simulink subsystem "test_actuation_system"  (R2021a)
settings: Solver=VariableStepAuto  StartTime=0.0  StopTime=10.0  RelTol=1e-3
libraries: sm_lib x51, nesl_utility x5
settings Model: Creator=Daniel Adejumo  LastModifiedBy=Daniel Adejumo

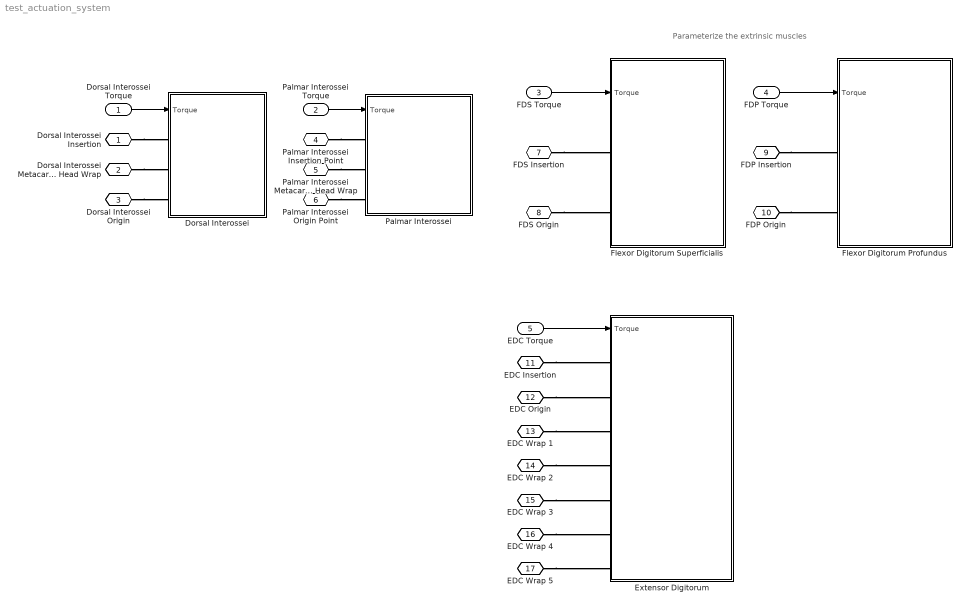
== system test_actuation_system ==
  note: Parameterize the extrinsic muscles
  Dorsal Interossei Torque : Inport
  Palmar Interossei Torque : Inport  Port=2
  FDS Torque : Inport  Port=3
  FDP Torque : Inport  Port=4
  EDC Torque : Inport  Port=5
  Dorsal Interossei : Subsystem
  Extensor Digitorum : Subsystem
  Flexor Digitorum Profundus : Subsystem
  Flexor Digitorum Superficialis : Subsystem
  Palmar Interossei : Subsystem
  Dorsal Interossei Insertion : PMIOPort  Side=Left
  Dorsal Interossei Metacarpal Head Wrap : PMIOPort  Port=2  Side=Left
  Dorsal Interossei Origin : PMIOPort  Port=3  Side=Left
  Palmar Interossei Insertion Point : PMIOPort  Port=4  Side=Left
  Palmar Interossei Metacarpal Head Wrap : PMIOPort  Port=5  Side=Left
  Palmar Interossei Origin Point : PMIOPort  Port=6  Side=Left
  FDS Insertion : PMIOPort  Port=7  Side=Left
  FDS Origin : PMIOPort  Port=8  Side=Left
  FDP Insertion : PMIOPort  Port=9  Side=Left
  FDP Origin : PMIOPort  Port=10  Side=Left
  EDC Insertion : PMIOPort  Port=11  Side=Left
  EDC Origin : PMIOPort  Port=12  Side=Left
  EDC Wrap 1 : PMIOPort  Port=13  Side=Left
  EDC Wrap 2 : PMIOPort  Port=14  Side=Left
  EDC Wrap 3 : PMIOPort  Port=15  Side=Left
  EDC Wrap 4 : PMIOPort  Port=16  Side=Left
  EDC Wrap 5 : PMIOPort  Port=17  Side=Left
  wires:
  Dorsal Interossei Torque/1 -> Dorsal Interossei/1(Torque)
  Palmar Interossei Torque/1 -> Palmar Interossei/1(Torque)
  FDS Torque/1 -> Flexor Digitorum Superficialis/1(Torque)
  FDP Torque/1 -> Flexor Digitorum Profundus/1(Torque)
  EDC Torque/1 -> Extensor Digitorum/1(Torque)
  connections:
  Dorsal Interossei Insertion/RConn1 -- Dorsal Interossei/LConn1
  Dorsal Interossei Metacarpal Head Wrap/RConn1 -- Dorsal Interossei/LConn2
  Dorsal Interossei Origin/RConn1 -- Dorsal Interossei/LConn3
  Palmar Interossei Insertion Point/RConn1 -- Palmar Interossei/LConn1
  FDS Insertion/RConn1 -- Flexor Digitorum Superficialis/LConn1
  FDS Origin/RConn1 -- Flexor Digitorum Superficialis/LConn2
  Palmar Interossei Metacarpal Head Wrap/RConn1 -- Palmar Interossei/LConn2
  Palmar Interossei Origin Point/RConn1 -- Palmar Interossei/LConn3
  FDP Origin/RConn1 -- Flexor Digitorum Profundus/LConn2
  FDP Insertion/RConn1 -- Flexor Digitorum Profundus/LConn1
  EDC Insertion/RConn1 -- Extensor Digitorum/LConn1
  EDC Origin/RConn1 -- Extensor Digitorum/LConn2
  EDC Wrap 1/RConn1 -- Extensor Digitorum/LConn3
  EDC Wrap 2/RConn1 -- Extensor Digitorum/LConn4
  EDC Wrap 3/RConn1 -- Extensor Digitorum/LConn5
  EDC Wrap 4/RConn1 -- Extensor Digitorum/LConn6
  EDC Wrap 5/RConn1 -- Extensor Digitorum/LConn7

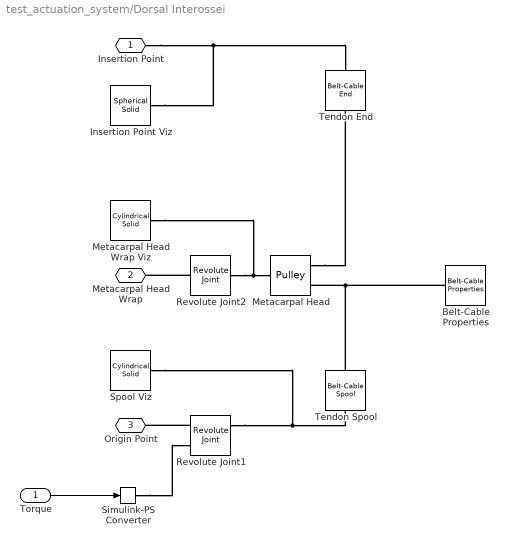
== system test_actuation_system/Dorsal Interossei ==
  Torque : Inport
  Belt-Cable Properties : sm_lib/Belts and Cables/Belt-Cable Properties  DrumBeltCableAlignment=Unrestricted  GraphicType=PitchLine  GraphicVisPropType=SimpleVisualProperties  GraphicDiffuseColor=viz.d2.dorsal_interossei.tendon_color  GraphicSpecularColor=[0.5 0.5 0.5 1.0]  GraphicAmbientColor=[0.15 0.15 0.15 1.0]  GraphicEmissiveColor=[0.0 0.0 0.0 1.0]  GraphicShininess=75  GraphicOpacity=viz.d2.dorsal_interossei.tendon_opacity
      settings: SourceProductBaseCode=MS
  Insertion Point Viz : sm_lib/Body Elements/Spherical Solid  GraphicAmbientColor=[0.15 0.15 0.15 1.0]  BasedOnType=Density  CenterOfMass=[0 0 0]  CenterOfMassUnits=m  GraphicDiffuseColor=viz.d2.dorsal_interossei.insertion_point_color  Density=dnm.link_density  DensityUnits=kg/m^3  DoExposeReferenceFrame=on  GraphicEmissiveColor=[0.0 0.0 0.0 1.0]  ExportEntireGeometry=off  SerializedExposedGeometries=<ExposedGeometries/>  SerializedFrames=<Frames/>  MarkerShape=Sphere  MarkerSize=10  GraphicType=FromGeometry  InertiaType=CalculateFromGeometry  Mass=1  MassUnits=kg  MomentsOfInertia=[1 1 1]  MomentsOfInertiaUnits=kg*m^2  GraphicOpacity=viz.d2.dorsal_interossei.insertion_point_opacity  ProductsOfInertia=[0 0 0]  ProductsOfInertiaUnits=kg*m^2  GraphicShininess=75  GraphicSpecularColor=[0.5 0.5 0.5 1.0]  SphereRadius=viz.d2.dorsal_interossei.insertion_point_radius  SphereRadiusUnits=m  GraphicVisPropType=SimpleVisualProperties
  Metacarpal Head : sm_lib/Belts and Cables/Pulley  PitchRadius=knm.d2.dorsal_interossei.wrap_pulleys_radius  PitchRadiusUnits=m  InitialWrapAngleLowerBound=knm.d2.dorsal_interossei.initial_wrap_lower_bound  InitialWrapAngleLowerBoundUnits=deg  SenseWrapAngle=off  SensePulleyAngleA=off  SensePulleyAngleB=off  SenseFleetAngleA=off  SenseFleetAngleB=off
      settings: SourceProductBaseCode=MS
  Metacarpal Head Wrap Viz : sm_lib/Body Elements/Cylindrical Solid  GraphicAmbientColor=[0.15 0.15 0.15 1.0]  BasedOnType=Density  CenterOfMass=[0 0 0]  CenterOfMassUnits=m  GraphicDiffuseColor=viz.d2.dorsal_interossei.wrap_pulleys_color  CylinderLength=viz.d2.dorsal_interossei.wrap_pulleys_length  CylinderLengthUnits=m  CylinderRadius=knm.d2.dorsal_interossei.wrap_pulleys_radius  CylinderRadiusUnits=m  Density=dnm.link_density  DensityUnits=kg/m^3  DoExposeReferenceFrame=on  GraphicEmissiveColor=[0.0 0.0 0.0 1.0]  ExportEntireGeometry=off  SerializedFrames=<Frames/>  MarkerShape=Sphere  MarkerSize=10  GraphicType=FromGeometry  InertiaType=CalculateFromGeometry  Mass=1  MassUnits=kg  MomentsOfInertia=[1 1 1]  MomentsOfInertiaUnits=kg*m^2  GraphicOpacity=viz.d2.dorsal_interossei.wrap_pulleys_opacity  ProductsOfInertia=[0 0 0]  ProductsOfInertiaUnits=kg*m^2  GraphicShininess=75  GraphicSpecularColor=[0.5 0.5 0.5 1.0]  GraphicVisPropType=SimpleVisualProperties
  Revolute Joint1 : sm_lib/Joints/Revolute Joint  JointMode=Normal  SenseConstraintForce=off  SenseConstraintForceX=off  SenseConstraintForceY=off  SenseConstraintForceZ=off  SenseConstraintTorque=off  SenseConstraintTorqueX=off  SenseConstraintTorqueY=off  SenseConstraintTorqueZ=off  SenseTotalForce=off  SenseTotalForceX=off  SenseTotalForceY=off  SenseTotalForceZ=off  SenseTotalTorque=off  SenseTotalTorqueX=off  SenseTotalTorqueY=off  SenseTotalTorqueZ=off  CompositeWrenchDir=FollowerOnBase  CompositeWrenchFrame=BaseFrame  EquilibriumPosition=0  EquilibriumPositionUnits=deg  SpringStiffness=0  SpringStiffnessUnits=N*m/deg  DampingCoefficient=0  DampingCoefficientUnits=N*m/(deg/s)  TorqueActuationMode=InputTorque  MotionActuationMode=ComputedMotion  SensePosition=off  SenseVelocity=on  SenseAcceleration=off  SenseTorqueForce=off  SenseLowerLimitTorqueForce=off  SenseUpperLimitTorqueForce=off  LowerLimitSpecify=off  LowerLimitBound=-90  LowerLimitBoundUnits=deg  LowerLimitStiffness=1e4  LowerLimitStiffnessUnits=N*m/deg  LowerLimitDamping=10  LowerLimitDampingUnits=N*m/(deg/s)  LowerLimitTransitionRegionWidth=0.1  LowerLimitTransitionRegionWidthUnits=deg  UpperLimitSpecify=off  UpperLimitBound=90  UpperLimitBoundUnits=deg  UpperLimitStiffness=1e4  UpperLimitStiffnessUnits=N*m/deg  UpperLimitDamping=10  UpperLimitDampingUnits=N*m/(deg/s)  UpperLimitTransitionRegionWidth=0.1  UpperLimitTransitionRegionWidthUnits=deg  PositionTargetSpecify=off  PositionTargetPriority=High  PositionTargetValue=0  PositionTargetValueUnits=deg  VelocityTargetSpecify=off  VelocityTargetPriority=High  VelocityTargetValue=0  VelocityTargetValueUnits=deg/s
  Revolute Joint2 : sm_lib/Joints/Revolute Joint  JointMode=Normal  SenseConstraintForce=off  SenseConstraintForceX=off  SenseConstraintForceY=off  SenseConstraintForceZ=off  SenseConstraintTorque=off  SenseConstraintTorqueX=off  SenseConstraintTorqueY=off  SenseConstraintTorqueZ=off  SenseTotalForce=off  SenseTotalForceX=off  SenseTotalForceY=off  SenseTotalForceZ=off  SenseTotalTorque=off  SenseTotalTorqueX=off  SenseTotalTorqueY=off  SenseTotalTorqueZ=off  CompositeWrenchDir=FollowerOnBase  CompositeWrenchFrame=BaseFrame  EquilibriumPosition=0  EquilibriumPositionUnits=deg  SpringStiffness=0  SpringStiffnessUnits=N*m/deg  DampingCoefficient=0  DampingCoefficientUnits=N*m/(deg/s)  TorqueActuationMode=NoTorque  MotionActuationMode=ComputedMotion  SensePosition=off  SenseVelocity=off  SenseAcceleration=off  SenseTorqueForce=off  SenseLowerLimitTorqueForce=off  SenseUpperLimitTorqueForce=off  LowerLimitSpecify=off  LowerLimitBound=-90  LowerLimitBoundUnits=deg  LowerLimitStiffness=1e4  LowerLimitStiffnessUnits=N*m/deg  LowerLimitDamping=10  LowerLimitDampingUnits=N*m/(deg/s)  LowerLimitTransitionRegionWidth=0.1  LowerLimitTransitionRegionWidthUnits=deg  UpperLimitSpecify=off  UpperLimitBound=90  UpperLimitBoundUnits=deg  UpperLimitStiffness=1e4  UpperLimitStiffnessUnits=N*m/deg  UpperLimitDamping=10  UpperLimitDampingUnits=N*m/(deg/s)  UpperLimitTransitionRegionWidth=0.1  UpperLimitTransitionRegionWidthUnits=deg  PositionTargetSpecify=off  PositionTargetPriority=High  PositionTargetValue=0  PositionTargetValueUnits=deg  VelocityTargetSpecify=off  VelocityTargetPriority=High  VelocityTargetValue=0  VelocityTargetValueUnits=deg/s
  Simulink-PS Converter : nesl_utility/Simulink-PS Converter  PhysicalDomain=network_engine_domain  SubClassName=ps_input  LeftPortType=input  RightPortType=output  PseudoPeriodic=off  Frequencies=[]  NoiseDistribution=none  NoiseParameters=[]  Unit=N*m  AffineConversion=off  FilteringAndDerivatives=filter  SimscapeFilterOrder=2  InputFilterTimeConstant=0.001  UdotUserProvided=0
      settings: SourceProductBaseCode=PW,SS
  Spool Viz : sm_lib/Body Elements/Cylindrical Solid  GraphicAmbientColor=[0.15 0.15 0.15 1.0]  BasedOnType=Density  CenterOfMass=[0 0 0]  CenterOfMassUnits=m  GraphicDiffuseColor=viz.d2.dorsal_interossei.spool_color  CylinderLength=viz.d2.dorsal_interossei.spool_length  CylinderLengthUnits=m  CylinderRadius=knm.d2.dorsal_interossei.pitch_radius  CylinderRadiusUnits=m  Density=dnm.link_density  DensityUnits=kg/m^3  DoExposeReferenceFrame=on  GraphicEmissiveColor=[0.0 0.0 0.0 1.0]  ExportEntireGeometry=off  SerializedFrames=<Frames/>  MarkerShape=Sphere  MarkerSize=10  GraphicType=FromGeometry  InertiaType=CalculateFromGeometry  Mass=1  MassUnits=kg  MomentsOfInertia=[1 1 1]  MomentsOfInertiaUnits=kg*m^2  GraphicOpacity=viz.d2.dorsal_interossei.spool_opacity  ProductsOfInertia=[0 0 0]  ProductsOfInertiaUnits=kg*m^2  GraphicShininess=75  GraphicSpecularColor=[0.5 0.5 0.5 1.0]  GraphicVisPropType=SimpleVisualProperties
  Tendon End : sm_lib/Belts and Cables/Belt-Cable End
      settings: SourceProductBaseCode=MS
  Tendon Spool : sm_lib/Belts and Cables/Belt-Cable Spool  PitchRadius=knm.d2.dorsal_interossei.pitch_radius  PitchRadiusUnits=m  SenseSpoolAngleA=off  SenseFleetAngleA=off
      settings: SourceProductBaseCode=MS
  Insertion Point : PMIOPort  Side=Left
  Metacarpal Head Wrap : PMIOPort  Port=2  Side=Left
  Origin Point : PMIOPort  Port=3  Side=Left
  wires:
  Torque/1 -> Simulink-PS Converter/1
  connections:
  Simulink-PS Converter/RConn1 -- Revolute Joint1/LConn2
  Metacarpal Head Wrap Viz/RConn1 -- Revolute Joint2/RConn1 -- Metacarpal Head/LConn1
  Revolute Joint2/LConn1 -- Metacarpal Head Wrap/RConn1
  Spool Viz/RConn1 -- Revolute Joint1/RConn1 -- Tendon Spool/LConn1
  Metacarpal Head/RConn1 -- Tendon End/RConn1
  Revolute Joint1/LConn1 -- Origin Point/RConn1
  Belt-Cable Properties/LConn1 -- Tendon Spool/RConn1 -- Metacarpal Head/RConn2
  Insertion Point Viz/RConn1 -- Insertion Point/RConn1 -- Tendon End/LConn1

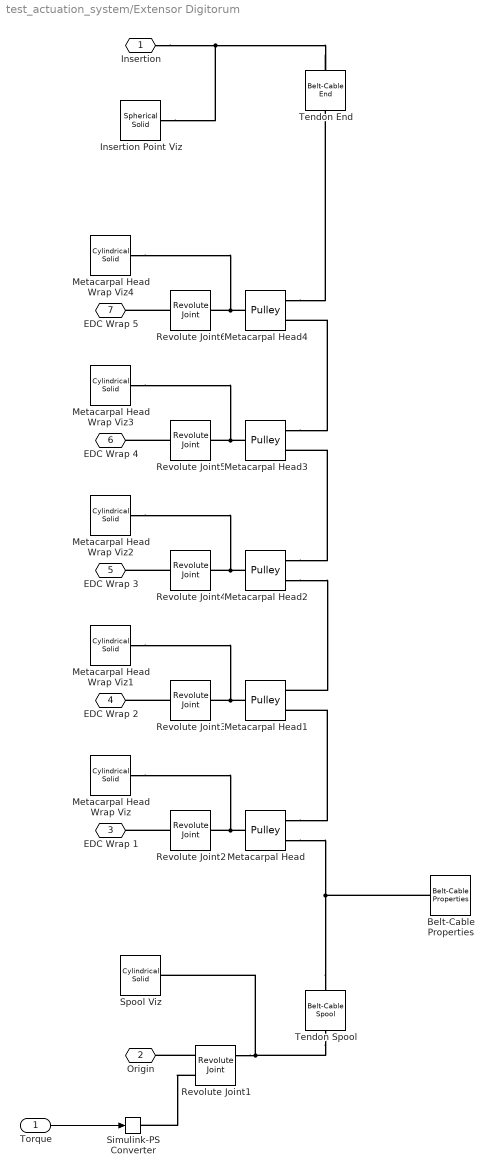
== system test_actuation_system/Extensor Digitorum ==
  Torque : Inport
  Belt-Cable Properties : sm_lib/Belts and Cables/Belt-Cable Properties  DrumBeltCableAlignment=Unrestricted  GraphicType=PitchLine  GraphicVisPropType=SimpleVisualProperties  GraphicDiffuseColor=viz.d2.palmar_interossei.tendon_color  GraphicSpecularColor=[0.5 0.5 0.5 1.0]  GraphicAmbientColor=[0.15 0.15 0.15 1.0]  GraphicEmissiveColor=[0.0 0.0 0.0 1.0]  GraphicShininess=75  GraphicOpacity=viz.d2.palmar_interossei.wrap_pulleys_opacity
      settings: SourceProductBaseCode=MS
  Insertion Point Viz : sm_lib/Body Elements/Spherical Solid  GraphicAmbientColor=[0.15 0.15 0.15 1.0]  BasedOnType=Density  CenterOfMass=[0 0 0]  CenterOfMassUnits=m  GraphicDiffuseColor=viz.d2.palmar_interossei.insertion_point_color  Density=1000  DensityUnits=kg/m^3  DoExposeReferenceFrame=on  GraphicEmissiveColor=[0.0 0.0 0.0 1.0]  ExportEntireGeometry=off  SerializedExposedGeometries=<ExposedGeometries/>  SerializedFrames=<Frames/>  MarkerShape=Sphere  MarkerSize=10  GraphicType=FromGeometry  InertiaType=CalculateFromGeometry  Mass=1  MassUnits=kg  MomentsOfInertia=[1 1 1]  MomentsOfInertiaUnits=kg*m^2  GraphicOpacity=viz.d2.palmar_interossei.insertion_point_opacity  ProductsOfInertia=[0 0 0]  ProductsOfInertiaUnits=kg*m^2  GraphicShininess=75  GraphicSpecularColor=[0.5 0.5 0.5 1.0]  SphereRadius=viz.d2.palmar_interossei.insertion_point_radius  SphereRadiusUnits=m  GraphicVisPropType=SimpleVisualProperties
  Metacarpal Head{,1..4} (5 alike) : sm_lib/Belts and Cables/Pulley  PitchRadius=knm.d2.palmar_interossei.wrap_pulleys_radius  PitchRadiusUnits=m  InitialWrapAngleLowerBound=knm.d2.palmar_interossei.initial_wrap_lower_bound  InitialWrapAngleLowerBoundUnits=deg  SenseWrapAngle=off  SensePulleyAngleA=off  SensePulleyAngleB=off  SenseFleetAngleA=off  SenseFleetAngleB=off
      settings: SourceProductBaseCode=MS
  Metacarpal Head Wrap Viz{,1..4} (5 alike) : sm_lib/Body Elements/Cylindrical Solid  GraphicAmbientColor=[0.15 0.15 0.15 1.0]  BasedOnType=Density  CenterOfMass=[0 0 0]  CenterOfMassUnits=m  GraphicDiffuseColor=viz.d2.palmar_interossei.wrap_pulleys_color  CylinderLength=viz.d2.palmar_interossei.wrap_pulleys_length  CylinderLengthUnits=m  CylinderRadius=knm.d2.palmar_interossei.wrap_pulleys_radius  CylinderRadiusUnits=m  Density=dnm.link_density  DensityUnits=kg/m^3  DoExposeReferenceFrame=on  GraphicEmissiveColor=[0.0 0.0 0.0 1.0]  ExportEntireGeometry=off  SerializedFrames=<Frames/>  MarkerShape=Sphere  MarkerSize=10  GraphicType=FromGeometry  InertiaType=CalculateFromGeometry  Mass=1  MassUnits=kg  MomentsOfInertia=[1 1 1]  MomentsOfInertiaUnits=kg*m^2  GraphicOpacity=viz.d2.palmar_interossei.wrap_pulleys_opacity  ProductsOfInertia=[0 0 0]  ProductsOfInertiaUnits=kg*m^2  GraphicShininess=75  GraphicSpecularColor=[0.5 0.5 0.5 1.0]  GraphicVisPropType=SimpleVisualProperties
  Revolute Joint1 : sm_lib/Joints/Revolute Joint  JointMode=Normal  SenseConstraintForce=off  SenseConstraintForceX=off  SenseConstraintForceY=off  SenseConstraintForceZ=off  SenseConstraintTorque=off  SenseConstraintTorqueX=off  SenseConstraintTorqueY=off  SenseConstraintTorqueZ=off  SenseTotalForce=off  SenseTotalForceX=off  SenseTotalForceY=off  SenseTotalForceZ=off  SenseTotalTorque=off  SenseTotalTorqueX=off  SenseTotalTorqueY=off  SenseTotalTorqueZ=off  CompositeWrenchDir=FollowerOnBase  CompositeWrenchFrame=BaseFrame  EquilibriumPosition=0  EquilibriumPositionUnits=deg  SpringStiffness=0  SpringStiffnessUnits=N*m/deg  DampingCoefficient=0  DampingCoefficientUnits=N*m/(deg/s)  TorqueActuationMode=InputTorque  MotionActuationMode=ComputedMotion  SensePosition=off  SenseVelocity=on  SenseAcceleration=off  SenseTorqueForce=off  SenseLowerLimitTorqueForce=off  SenseUpperLimitTorqueForce=off  LowerLimitSpecify=off  LowerLimitBound=-90  LowerLimitBoundUnits=deg  LowerLimitStiffness=1e4  LowerLimitStiffnessUnits=N*m/deg  LowerLimitDamping=10  LowerLimitDampingUnits=N*m/(deg/s)  LowerLimitTransitionRegionWidth=0.1  LowerLimitTransitionRegionWidthUnits=deg  UpperLimitSpecify=off  UpperLimitBound=90  UpperLimitBoundUnits=deg  UpperLimitStiffness=1e4  UpperLimitStiffnessUnits=N*m/deg  UpperLimitDamping=10  UpperLimitDampingUnits=N*m/(deg/s)  UpperLimitTransitionRegionWidth=0.1  UpperLimitTransitionRegionWidthUnits=deg  PositionTargetSpecify=off  PositionTargetPriority=High  PositionTargetValue=0  PositionTargetValueUnits=deg  VelocityTargetSpecify=off  VelocityTargetPriority=High  VelocityTargetValue=0  VelocityTargetValueUnits=deg/s
  Revolute Joint{2..6} (5 alike) : sm_lib/Joints/Revolute Joint  JointMode=Normal  SenseConstraintForce=off  SenseConstraintForceX=off  SenseConstraintForceY=off  SenseConstraintForceZ=off  SenseConstraintTorque=off  SenseConstraintTorqueX=off  SenseConstraintTorqueY=off  SenseConstraintTorqueZ=off  SenseTotalForce=off  SenseTotalForceX=off  SenseTotalForceY=off  SenseTotalForceZ=off  SenseTotalTorque=off  SenseTotalTorqueX=off  SenseTotalTorqueY=off  SenseTotalTorqueZ=off  CompositeWrenchDir=FollowerOnBase  CompositeWrenchFrame=BaseFrame  EquilibriumPosition=0  EquilibriumPositionUnits=deg  SpringStiffness=0  SpringStiffnessUnits=N*m/deg  DampingCoefficient=0  DampingCoefficientUnits=N*m/(deg/s)  TorqueActuationMode=NoTorque  MotionActuationMode=ComputedMotion  SensePosition=off  SenseVelocity=off  SenseAcceleration=off  SenseTorqueForce=off  SenseLowerLimitTorqueForce=off  SenseUpperLimitTorqueForce=off  LowerLimitSpecify=off  LowerLimitBound=-90  LowerLimitBoundUnits=deg  LowerLimitStiffness=1e4  LowerLimitStiffnessUnits=N*m/deg  LowerLimitDamping=10  LowerLimitDampingUnits=N*m/(deg/s)  LowerLimitTransitionRegionWidth=0.1  LowerLimitTransitionRegionWidthUnits=deg  UpperLimitSpecify=off  UpperLimitBound=90  UpperLimitBoundUnits=deg  UpperLimitStiffness=1e4  UpperLimitStiffnessUnits=N*m/deg  UpperLimitDamping=10  UpperLimitDampingUnits=N*m/(deg/s)  UpperLimitTransitionRegionWidth=0.1  UpperLimitTransitionRegionWidthUnits=deg  PositionTargetSpecify=off  PositionTargetPriority=High  PositionTargetValue=0  PositionTargetValueUnits=deg  VelocityTargetSpecify=off  VelocityTargetPriority=High  VelocityTargetValue=0  VelocityTargetValueUnits=deg/s
  Simulink-PS Converter : nesl_utility/Simulink-PS Converter  PhysicalDomain=network_engine_domain  SubClassName=ps_input  LeftPortType=input  RightPortType=output  PseudoPeriodic=off  Frequencies=[]  NoiseDistribution=none  NoiseParameters=[]  Unit=N*m  AffineConversion=off  FilteringAndDerivatives=filter  SimscapeFilterOrder=2  InputFilterTimeConstant=0.001  UdotUserProvided=0
      settings: SourceProductBaseCode=PW,SS
  Spool Viz : sm_lib/Body Elements/Cylindrical Solid  GraphicAmbientColor=[0.15 0.15 0.15 1.0]  BasedOnType=Density  CenterOfMass=[0 0 0]  CenterOfMassUnits=m  GraphicDiffuseColor=viz.d2.palmar_interossei.spool_color  CylinderLength=viz.d2.palmar_interossei.spool_length  CylinderLengthUnits=m  CylinderRadius=knm.d2.palmar_interossei.pitch_radius  CylinderRadiusUnits=m  Density=dnm.link_density  DensityUnits=kg/m^3  DoExposeReferenceFrame=on  GraphicEmissiveColor=[0.0 0.0 0.0 1.0]  ExportEntireGeometry=off  SerializedFrames=<Frames/>  MarkerShape=Sphere  MarkerSize=10  GraphicType=FromGeometry  InertiaType=CalculateFromGeometry  Mass=1  MassUnits=kg  MomentsOfInertia=[1 1 1]  MomentsOfInertiaUnits=kg*m^2  GraphicOpacity=viz.d2.palmar_interossei.spool_opacity  ProductsOfInertia=[0 0 0]  ProductsOfInertiaUnits=kg*m^2  GraphicShininess=75  GraphicSpecularColor=[0.5 0.5 0.5 1.0]  GraphicVisPropType=SimpleVisualProperties
  Tendon End : sm_lib/Belts and Cables/Belt-Cable End
      settings: SourceProductBaseCode=MS
  Tendon Spool : sm_lib/Belts and Cables/Belt-Cable Spool  PitchRadius=knm.d2.palmar_interossei.pitch_radius  PitchRadiusUnits=m  SenseSpoolAngleA=off  SenseFleetAngleA=off
      settings: SourceProductBaseCode=MS
  Insertion : PMIOPort  Side=Left
  Origin : PMIOPort  Port=2  Side=Left
  EDC Wrap 1 : PMIOPort  Port=3  Side=Left
  EDC Wrap 2 : PMIOPort  Port=4  Side=Left
  EDC Wrap 3 : PMIOPort  Port=5  Side=Left
  EDC Wrap 4 : PMIOPort  Port=6  Side=Left
  EDC Wrap 5 : PMIOPort  Port=7  Side=Left
  wires:
  Torque/1 -> Simulink-PS Converter/1
  connections:
  Metacarpal Head4/RConn1 -- Tendon End/RConn1
  Metacarpal Head3/RConn1 -- Metacarpal Head4/RConn2
  Metacarpal Head2/RConn1 -- Metacarpal Head3/RConn2
  Metacarpal Head2/RConn2 -- Metacarpal Head1/RConn1
  Metacarpal Head/RConn1 -- Metacarpal Head1/RConn2
  Revolute Joint6/LConn1 -- EDC Wrap 5/RConn1
  Revolute Joint6/RConn1 -- Metacarpal Head Wrap Viz4/RConn1 -- Metacarpal Head4/LConn1
  Revolute Joint5/LConn1 -- EDC Wrap 4/RConn1
  Metacarpal Head Wrap Viz3/RConn1 -- Revolute Joint5/RConn1 -- Metacarpal Head3/LConn1
  Revolute Joint4/LConn1 -- EDC Wrap 3/RConn1
  Revolute Joint4/RConn1 -- Metacarpal Head Wrap Viz2/RConn1 -- Metacarpal Head2/LConn1
  Revolute Joint3/LConn1 -- EDC Wrap 2/RConn1
  Metacarpal Head Wrap Viz1/RConn1 -- Revolute Joint3/RConn1 -- Metacarpal Head1/LConn1
  Revolute Joint2/LConn1 -- EDC Wrap 1/RConn1
  Revolute Joint2/RConn1 -- Metacarpal Head Wrap Viz/RConn1 -- Metacarpal Head/LConn1
  Revolute Joint1/LConn1 -- Origin/RConn1
  Revolute Joint1/LConn2 -- Simulink-PS Converter/RConn1
  Revolute Joint1/RConn1 -- Spool Viz/RConn1 -- Tendon Spool/LConn1
  Tendon Spool/RConn1 -- Belt-Cable Properties/LConn1 -- Metacarpal Head/RConn2
  Tendon End/LConn1 -- Insertion/RConn1 -- Insertion Point Viz/RConn1

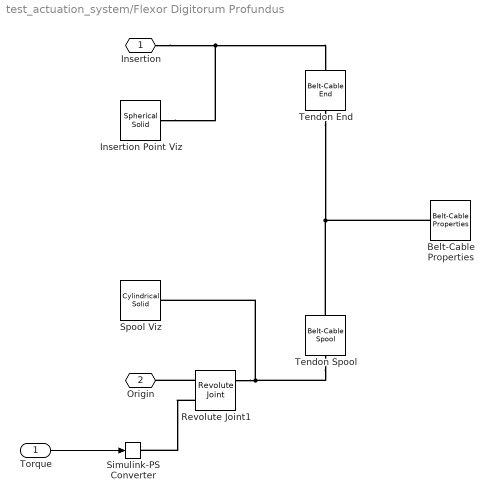
== system test_actuation_system/Flexor Digitorum Profundus ==
  Torque : Inport
  Belt-Cable Properties : sm_lib/Belts and Cables/Belt-Cable Properties  DrumBeltCableAlignment=Unrestricted  GraphicType=PitchLine  GraphicVisPropType=SimpleVisualProperties  GraphicDiffuseColor=viz.d2.palmar_interossei.tendon_color  GraphicSpecularColor=[0.5 0.5 0.5 1.0]  GraphicAmbientColor=[0.15 0.15 0.15 1.0]  GraphicEmissiveColor=[0.0 0.0 0.0 1.0]  GraphicShininess=75  GraphicOpacity=viz.d2.palmar_interossei.wrap_pulleys_opacity
      settings: SourceProductBaseCode=MS
  Insertion Point Viz : sm_lib/Body Elements/Spherical Solid  GraphicAmbientColor=[0.15 0.15 0.15 1.0]  BasedOnType=Density  CenterOfMass=[0 0 0]  CenterOfMassUnits=m  GraphicDiffuseColor=viz.d2.palmar_interossei.insertion_point_color  Density=1000  DensityUnits=kg/m^3  DoExposeReferenceFrame=on  GraphicEmissiveColor=[0.0 0.0 0.0 1.0]  ExportEntireGeometry=off  SerializedExposedGeometries=<ExposedGeometries/>  SerializedFrames=<Frames/>  MarkerShape=Sphere  MarkerSize=10  GraphicType=FromGeometry  InertiaType=CalculateFromGeometry  Mass=1  MassUnits=kg  MomentsOfInertia=[1 1 1]  MomentsOfInertiaUnits=kg*m^2  GraphicOpacity=viz.d2.palmar_interossei.insertion_point_opacity  ProductsOfInertia=[0 0 0]  ProductsOfInertiaUnits=kg*m^2  GraphicShininess=75  GraphicSpecularColor=[0.5 0.5 0.5 1.0]  SphereRadius=viz.d2.palmar_interossei.insertion_point_radius  SphereRadiusUnits=m  GraphicVisPropType=SimpleVisualProperties
  Revolute Joint1 : sm_lib/Joints/Revolute Joint  JointMode=Normal  SenseConstraintForce=off  SenseConstraintForceX=off  SenseConstraintForceY=off  SenseConstraintForceZ=off  SenseConstraintTorque=off  SenseConstraintTorqueX=off  SenseConstraintTorqueY=off  SenseConstraintTorqueZ=off  SenseTotalForce=off  SenseTotalForceX=off  SenseTotalForceY=off  SenseTotalForceZ=off  SenseTotalTorque=off  SenseTotalTorqueX=off  SenseTotalTorqueY=off  SenseTotalTorqueZ=off  CompositeWrenchDir=FollowerOnBase  CompositeWrenchFrame=BaseFrame  EquilibriumPosition=0  EquilibriumPositionUnits=deg  SpringStiffness=0  SpringStiffnessUnits=N*m/deg  DampingCoefficient=0  DampingCoefficientUnits=N*m/(deg/s)  TorqueActuationMode=InputTorque  MotionActuationMode=ComputedMotion  SensePosition=off  SenseVelocity=on  SenseAcceleration=off  SenseTorqueForce=off  SenseLowerLimitTorqueForce=off  SenseUpperLimitTorqueForce=off  LowerLimitSpecify=off  LowerLimitBound=-90  LowerLimitBoundUnits=deg  LowerLimitStiffness=1e4  LowerLimitStiffnessUnits=N*m/deg  LowerLimitDamping=10  LowerLimitDampingUnits=N*m/(deg/s)  LowerLimitTransitionRegionWidth=0.1  LowerLimitTransitionRegionWidthUnits=deg  UpperLimitSpecify=off  UpperLimitBound=90  UpperLimitBoundUnits=deg  UpperLimitStiffness=1e4  UpperLimitStiffnessUnits=N*m/deg  UpperLimitDamping=10  UpperLimitDampingUnits=N*m/(deg/s)  UpperLimitTransitionRegionWidth=0.1  UpperLimitTransitionRegionWidthUnits=deg  PositionTargetSpecify=off  PositionTargetPriority=High  PositionTargetValue=0  PositionTargetValueUnits=deg  VelocityTargetSpecify=off  VelocityTargetPriority=High  VelocityTargetValue=0  VelocityTargetValueUnits=deg/s
  Simulink-PS Converter : nesl_utility/Simulink-PS Converter  PhysicalDomain=network_engine_domain  SubClassName=ps_input  LeftPortType=input  RightPortType=output  PseudoPeriodic=off  Frequencies=[]  NoiseDistribution=none  NoiseParameters=[]  Unit=N*m  AffineConversion=off  FilteringAndDerivatives=filter  SimscapeFilterOrder=2  InputFilterTimeConstant=0.001  UdotUserProvided=0
      settings: SourceProductBaseCode=PW,SS
  Spool Viz : sm_lib/Body Elements/Cylindrical Solid  GraphicAmbientColor=[0.15 0.15 0.15 1.0]  BasedOnType=Density  CenterOfMass=[0 0 0]  CenterOfMassUnits=m  GraphicDiffuseColor=viz.d2.palmar_interossei.spool_color  CylinderLength=viz.d2.palmar_interossei.spool_length  CylinderLengthUnits=m  CylinderRadius=knm.d2.palmar_interossei.pitch_radius  CylinderRadiusUnits=m  Density=dnm.link_density  DensityUnits=kg/m^3  DoExposeReferenceFrame=on  GraphicEmissiveColor=[0.0 0.0 0.0 1.0]  ExportEntireGeometry=off  SerializedFrames=<Frames/>  MarkerShape=Sphere  MarkerSize=10  GraphicType=FromGeometry  InertiaType=CalculateFromGeometry  Mass=1  MassUnits=kg  MomentsOfInertia=[1 1 1]  MomentsOfInertiaUnits=kg*m^2  GraphicOpacity=viz.d2.palmar_interossei.spool_opacity  ProductsOfInertia=[0 0 0]  ProductsOfInertiaUnits=kg*m^2  GraphicShininess=75  GraphicSpecularColor=[0.5 0.5 0.5 1.0]  GraphicVisPropType=SimpleVisualProperties
  Tendon End : sm_lib/Belts and Cables/Belt-Cable End
      settings: SourceProductBaseCode=MS
  Tendon Spool : sm_lib/Belts and Cables/Belt-Cable Spool  PitchRadius=knm.d2.palmar_interossei.pitch_radius  PitchRadiusUnits=m  SenseSpoolAngleA=off  SenseFleetAngleA=off
      settings: SourceProductBaseCode=MS
  Insertion : PMIOPort  Side=Left
  Origin : PMIOPort  Port=2  Side=Left
  wires:
  Torque/1 -> Simulink-PS Converter/1
  connections:
  Insertion Point Viz/RConn1 -- Insertion/RConn1 -- Tendon End/LConn1
  Tendon Spool/RConn1 -- Tendon End/RConn1 -- Belt-Cable Properties/LConn1
  Tendon Spool/LConn1 -- Spool Viz/RConn1 -- Revolute Joint1/RConn1
  Revolute Joint1/LConn2 -- Simulink-PS Converter/RConn1
  Revolute Joint1/LConn1 -- Origin/RConn1

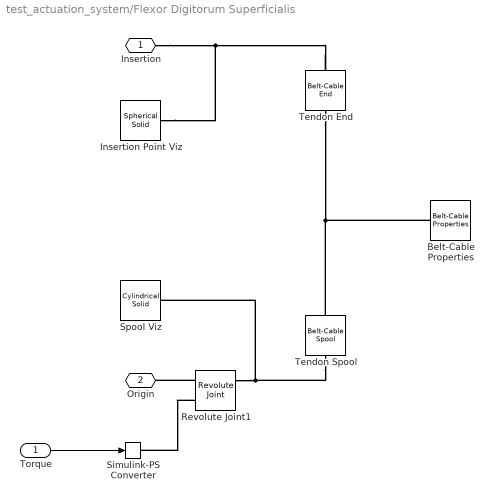
== system test_actuation_system/Flexor Digitorum Superficialis ==
  Torque : Inport
  Belt-Cable Properties : sm_lib/Belts and Cables/Belt-Cable Properties  DrumBeltCableAlignment=Unrestricted  GraphicType=PitchLine  GraphicVisPropType=SimpleVisualProperties  GraphicDiffuseColor=viz.d2.palmar_interossei.tendon_color  GraphicSpecularColor=[0.5 0.5 0.5 1.0]  GraphicAmbientColor=[0.15 0.15 0.15 1.0]  GraphicEmissiveColor=[0.0 0.0 0.0 1.0]  GraphicShininess=75  GraphicOpacity=viz.d2.palmar_interossei.wrap_pulleys_opacity
      settings: SourceProductBaseCode=MS
  Insertion Point Viz : sm_lib/Body Elements/Spherical Solid  GraphicAmbientColor=[0.15 0.15 0.15 1.0]  BasedOnType=Density  CenterOfMass=[0 0 0]  CenterOfMassUnits=m  GraphicDiffuseColor=viz.d2.palmar_interossei.insertion_point_color  Density=1000  DensityUnits=kg/m^3  DoExposeReferenceFrame=on  GraphicEmissiveColor=[0.0 0.0 0.0 1.0]  ExportEntireGeometry=off  SerializedExposedGeometries=<ExposedGeometries/>  SerializedFrames=<Frames/>  MarkerShape=Sphere  MarkerSize=10  GraphicType=FromGeometry  InertiaType=CalculateFromGeometry  Mass=1  MassUnits=kg  MomentsOfInertia=[1 1 1]  MomentsOfInertiaUnits=kg*m^2  GraphicOpacity=viz.d2.palmar_interossei.insertion_point_opacity  ProductsOfInertia=[0 0 0]  ProductsOfInertiaUnits=kg*m^2  GraphicShininess=75  GraphicSpecularColor=[0.5 0.5 0.5 1.0]  SphereRadius=viz.d2.palmar_interossei.insertion_point_radius  SphereRadiusUnits=m  GraphicVisPropType=SimpleVisualProperties
  Revolute Joint1 : sm_lib/Joints/Revolute Joint  JointMode=Normal  SenseConstraintForce=off  SenseConstraintForceX=off  SenseConstraintForceY=off  SenseConstraintForceZ=off  SenseConstraintTorque=off  SenseConstraintTorqueX=off  SenseConstraintTorqueY=off  SenseConstraintTorqueZ=off  SenseTotalForce=off  SenseTotalForceX=off  SenseTotalForceY=off  SenseTotalForceZ=off  SenseTotalTorque=off  SenseTotalTorqueX=off  SenseTotalTorqueY=off  SenseTotalTorqueZ=off  CompositeWrenchDir=FollowerOnBase  CompositeWrenchFrame=BaseFrame  EquilibriumPosition=0  EquilibriumPositionUnits=deg  SpringStiffness=0  SpringStiffnessUnits=N*m/deg  DampingCoefficient=0  DampingCoefficientUnits=N*m/(deg/s)  TorqueActuationMode=InputTorque  MotionActuationMode=ComputedMotion  SensePosition=off  SenseVelocity=on  SenseAcceleration=off  SenseTorqueForce=off  SenseLowerLimitTorqueForce=off  SenseUpperLimitTorqueForce=off  LowerLimitSpecify=off  LowerLimitBound=-90  LowerLimitBoundUnits=deg  LowerLimitStiffness=1e4  LowerLimitStiffnessUnits=N*m/deg  LowerLimitDamping=10  LowerLimitDampingUnits=N*m/(deg/s)  LowerLimitTransitionRegionWidth=0.1  LowerLimitTransitionRegionWidthUnits=deg  UpperLimitSpecify=off  UpperLimitBound=90  UpperLimitBoundUnits=deg  UpperLimitStiffness=1e4  UpperLimitStiffnessUnits=N*m/deg  UpperLimitDamping=10  UpperLimitDampingUnits=N*m/(deg/s)  UpperLimitTransitionRegionWidth=0.1  UpperLimitTransitionRegionWidthUnits=deg  PositionTargetSpecify=off  PositionTargetPriority=High  PositionTargetValue=0  PositionTargetValueUnits=deg  VelocityTargetSpecify=off  VelocityTargetPriority=High  VelocityTargetValue=0  VelocityTargetValueUnits=deg/s
  Simulink-PS Converter : nesl_utility/Simulink-PS Converter  PhysicalDomain=network_engine_domain  SubClassName=ps_input  LeftPortType=input  RightPortType=output  PseudoPeriodic=off  Frequencies=[]  NoiseDistribution=none  NoiseParameters=[]  Unit=N*m  AffineConversion=off  FilteringAndDerivatives=filter  SimscapeFilterOrder=2  InputFilterTimeConstant=0.001  UdotUserProvided=0
      settings: SourceProductBaseCode=PW,SS
  Spool Viz : sm_lib/Body Elements/Cylindrical Solid  GraphicAmbientColor=[0.15 0.15 0.15 1.0]  BasedOnType=Density  CenterOfMass=[0 0 0]  CenterOfMassUnits=m  GraphicDiffuseColor=viz.d2.palmar_interossei.spool_color  CylinderLength=viz.d2.palmar_interossei.spool_length  CylinderLengthUnits=m  CylinderRadius=knm.d2.palmar_interossei.pitch_radius  CylinderRadiusUnits=m  Density=dnm.link_density  DensityUnits=kg/m^3  DoExposeReferenceFrame=on  GraphicEmissiveColor=[0.0 0.0 0.0 1.0]  ExportEntireGeometry=off  SerializedFrames=<Frames/>  MarkerShape=Sphere  MarkerSize=10  GraphicType=FromGeometry  InertiaType=CalculateFromGeometry  Mass=1  MassUnits=kg  MomentsOfInertia=[1 1 1]  MomentsOfInertiaUnits=kg*m^2  GraphicOpacity=viz.d2.palmar_interossei.spool_opacity  ProductsOfInertia=[0 0 0]  ProductsOfInertiaUnits=kg*m^2  GraphicShininess=75  GraphicSpecularColor=[0.5 0.5 0.5 1.0]  GraphicVisPropType=SimpleVisualProperties
  Tendon End : sm_lib/Belts and Cables/Belt-Cable End
      settings: SourceProductBaseCode=MS
  Tendon Spool : sm_lib/Belts and Cables/Belt-Cable Spool  PitchRadius=knm.d2.palmar_interossei.pitch_radius  PitchRadiusUnits=m  SenseSpoolAngleA=off  SenseFleetAngleA=off
      settings: SourceProductBaseCode=MS
  Insertion : PMIOPort  Side=Left
  Origin : PMIOPort  Port=2  Side=Left
  wires:
  Torque/1 -> Simulink-PS Converter/1
  connections:
  Revolute Joint1/LConn1 -- Origin/RConn1
  Revolute Joint1/LConn2 -- Simulink-PS Converter/RConn1
  Revolute Joint1/RConn1 -- Spool Viz/RConn1 -- Tendon Spool/LConn1
  Belt-Cable Properties/LConn1 -- Tendon End/RConn1 -- Tendon Spool/RConn1
  Tendon End/LConn1 -- Insertion/RConn1 -- Insertion Point Viz/RConn1

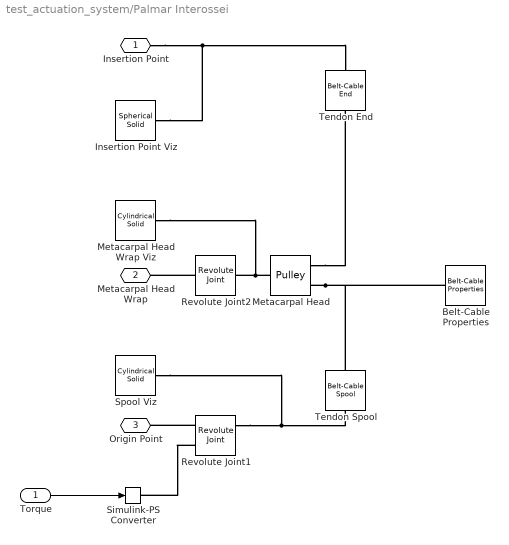
== system test_actuation_system/Palmar Interossei ==
  Torque : Inport
  Belt-Cable Properties : sm_lib/Belts and Cables/Belt-Cable Properties  DrumBeltCableAlignment=Unrestricted  GraphicType=PitchLine  GraphicVisPropType=SimpleVisualProperties  GraphicDiffuseColor=viz.d2.palmar_interossei.tendon_color  GraphicSpecularColor=[0.5 0.5 0.5 1.0]  GraphicAmbientColor=[0.15 0.15 0.15 1.0]  GraphicEmissiveColor=[0.0 0.0 0.0 1.0]  GraphicShininess=75  GraphicOpacity=viz.d2.palmar_interossei.wrap_pulleys_opacity
      settings: SourceProductBaseCode=MS
  Insertion Point Viz : sm_lib/Body Elements/Spherical Solid  GraphicAmbientColor=[0.15 0.15 0.15 1.0]  BasedOnType=Density  CenterOfMass=[0 0 0]  CenterOfMassUnits=m  GraphicDiffuseColor=viz.d2.palmar_interossei.insertion_point_color  Density=dnm.link_density  DensityUnits=kg/m^3  DoExposeReferenceFrame=on  GraphicEmissiveColor=[0.0 0.0 0.0 1.0]  ExportEntireGeometry=off  SerializedExposedGeometries=<ExposedGeometries/>  SerializedFrames=<Frames/>  MarkerShape=Sphere  MarkerSize=10  GraphicType=FromGeometry  InertiaType=CalculateFromGeometry  Mass=1  MassUnits=kg  MomentsOfInertia=[1 1 1]  MomentsOfInertiaUnits=kg*m^2  GraphicOpacity=viz.d2.palmar_interossei.insertion_point_opacity  ProductsOfInertia=[0 0 0]  ProductsOfInertiaUnits=kg*m^2  GraphicShininess=75  GraphicSpecularColor=[0.5 0.5 0.5 1.0]  SphereRadius=viz.d2.palmar_interossei.insertion_point_radius  SphereRadiusUnits=m  GraphicVisPropType=SimpleVisualProperties
  Metacarpal Head : sm_lib/Belts and Cables/Pulley  PitchRadius=knm.d2.palmar_interossei.wrap_pulleys_radius  PitchRadiusUnits=m  InitialWrapAngleLowerBound=knm.d2.palmar_interossei.initial_wrap_lower_bound  InitialWrapAngleLowerBoundUnits=deg  SenseWrapAngle=off  SensePulleyAngleA=off  SensePulleyAngleB=off  SenseFleetAngleA=off  SenseFleetAngleB=off
      settings: SourceProductBaseCode=MS
  Metacarpal Head Wrap Viz : sm_lib/Body Elements/Cylindrical Solid  GraphicAmbientColor=[0.15 0.15 0.15 1.0]  BasedOnType=Density  CenterOfMass=[0 0 0]  CenterOfMassUnits=m  GraphicDiffuseColor=viz.d2.palmar_interossei.wrap_pulleys_color  CylinderLength=viz.d2.palmar_interossei.wrap_pulleys_length  CylinderLengthUnits=m  CylinderRadius=knm.d2.palmar_interossei.wrap_pulleys_radius  CylinderRadiusUnits=m  Density=dnm.link_density  DensityUnits=kg/m^3  DoExposeReferenceFrame=on  GraphicEmissiveColor=[0.0 0.0 0.0 1.0]  ExportEntireGeometry=off  SerializedFrames=<Frames/>  MarkerShape=Sphere  MarkerSize=10  GraphicType=FromGeometry  InertiaType=CalculateFromGeometry  Mass=1  MassUnits=kg  MomentsOfInertia=[1 1 1]  MomentsOfInertiaUnits=kg*m^2  GraphicOpacity=viz.d2.palmar_interossei.wrap_pulleys_opacity  ProductsOfInertia=[0 0 0]  ProductsOfInertiaUnits=kg*m^2  GraphicShininess=75  GraphicSpecularColor=[0.5 0.5 0.5 1.0]  GraphicVisPropType=SimpleVisualProperties
  Revolute Joint1 : sm_lib/Joints/Revolute Joint  JointMode=Normal  SenseConstraintForce=off  SenseConstraintForceX=off  SenseConstraintForceY=off  SenseConstraintForceZ=off  SenseConstraintTorque=off  SenseConstraintTorqueX=off  SenseConstraintTorqueY=off  SenseConstraintTorqueZ=off  SenseTotalForce=off  SenseTotalForceX=off  SenseTotalForceY=off  SenseTotalForceZ=off  SenseTotalTorque=off  SenseTotalTorqueX=off  SenseTotalTorqueY=off  SenseTotalTorqueZ=off  CompositeWrenchDir=FollowerOnBase  CompositeWrenchFrame=BaseFrame  EquilibriumPosition=0  EquilibriumPositionUnits=deg  SpringStiffness=0  SpringStiffnessUnits=N*m/deg  DampingCoefficient=0  DampingCoefficientUnits=N*m/(deg/s)  TorqueActuationMode=InputTorque  MotionActuationMode=ComputedMotion  SensePosition=off  SenseVelocity=on  SenseAcceleration=off  SenseTorqueForce=off  SenseLowerLimitTorqueForce=off  SenseUpperLimitTorqueForce=off  LowerLimitSpecify=off  LowerLimitBound=-90  LowerLimitBoundUnits=deg  LowerLimitStiffness=1e4  LowerLimitStiffnessUnits=N*m/deg  LowerLimitDamping=10  LowerLimitDampingUnits=N*m/(deg/s)  LowerLimitTransitionRegionWidth=0.1  LowerLimitTransitionRegionWidthUnits=deg  UpperLimitSpecify=off  UpperLimitBound=90  UpperLimitBoundUnits=deg  UpperLimitStiffness=1e4  UpperLimitStiffnessUnits=N*m/deg  UpperLimitDamping=10  UpperLimitDampingUnits=N*m/(deg/s)  UpperLimitTransitionRegionWidth=0.1  UpperLimitTransitionRegionWidthUnits=deg  PositionTargetSpecify=off  PositionTargetPriority=High  PositionTargetValue=0  PositionTargetValueUnits=deg  VelocityTargetSpecify=off  VelocityTargetPriority=High  VelocityTargetValue=0  VelocityTargetValueUnits=deg/s
  Revolute Joint2 : sm_lib/Joints/Revolute Joint  JointMode=Normal  SenseConstraintForce=off  SenseConstraintForceX=off  SenseConstraintForceY=off  SenseConstraintForceZ=off  SenseConstraintTorque=off  SenseConstraintTorqueX=off  SenseConstraintTorqueY=off  SenseConstraintTorqueZ=off  SenseTotalForce=off  SenseTotalForceX=off  SenseTotalForceY=off  SenseTotalForceZ=off  SenseTotalTorque=off  SenseTotalTorqueX=off  SenseTotalTorqueY=off  SenseTotalTorqueZ=off  CompositeWrenchDir=FollowerOnBase  CompositeWrenchFrame=BaseFrame  EquilibriumPosition=0  EquilibriumPositionUnits=deg  SpringStiffness=0  SpringStiffnessUnits=N*m/deg  DampingCoefficient=0  DampingCoefficientUnits=N*m/(deg/s)  TorqueActuationMode=NoTorque  MotionActuationMode=ComputedMotion  SensePosition=off  SenseVelocity=off  SenseAcceleration=off  SenseTorqueForce=off  SenseLowerLimitTorqueForce=off  SenseUpperLimitTorqueForce=off  LowerLimitSpecify=off  LowerLimitBound=-90  LowerLimitBoundUnits=deg  LowerLimitStiffness=1e4  LowerLimitStiffnessUnits=N*m/deg  LowerLimitDamping=10  LowerLimitDampingUnits=N*m/(deg/s)  LowerLimitTransitionRegionWidth=0.1  LowerLimitTransitionRegionWidthUnits=deg  UpperLimitSpecify=off  UpperLimitBound=90  UpperLimitBoundUnits=deg  UpperLimitStiffness=1e4  UpperLimitStiffnessUnits=N*m/deg  UpperLimitDamping=10  UpperLimitDampingUnits=N*m/(deg/s)  UpperLimitTransitionRegionWidth=0.1  UpperLimitTransitionRegionWidthUnits=deg  PositionTargetSpecify=off  PositionTargetPriority=High  PositionTargetValue=0  PositionTargetValueUnits=deg  VelocityTargetSpecify=off  VelocityTargetPriority=High  VelocityTargetValue=0  VelocityTargetValueUnits=deg/s
  Simulink-PS Converter : nesl_utility/Simulink-PS Converter  PhysicalDomain=network_engine_domain  SubClassName=ps_input  LeftPortType=input  RightPortType=output  PseudoPeriodic=off  Frequencies=[]  NoiseDistribution=none  NoiseParameters=[]  Unit=N*m  AffineConversion=off  FilteringAndDerivatives=filter  SimscapeFilterOrder=2  InputFilterTimeConstant=0.001  UdotUserProvided=0
      settings: SourceProductBaseCode=PW,SS
  Spool Viz : sm_lib/Body Elements/Cylindrical Solid  GraphicAmbientColor=[0.15 0.15 0.15 1.0]  BasedOnType=Density  CenterOfMass=[0 0 0]  CenterOfMassUnits=m  GraphicDiffuseColor=viz.d2.palmar_interossei.spool_color  CylinderLength=viz.d2.palmar_interossei.spool_length  CylinderLengthUnits=m  CylinderRadius=knm.d2.palmar_interossei.pitch_radius  CylinderRadiusUnits=m  Density=dnm.link_density  DensityUnits=kg/m^3  DoExposeReferenceFrame=on  GraphicEmissiveColor=[0.0 0.0 0.0 1.0]  ExportEntireGeometry=off  SerializedFrames=<Frames/>  MarkerShape=Sphere  MarkerSize=10  GraphicType=FromGeometry  InertiaType=CalculateFromGeometry  Mass=1  MassUnits=kg  MomentsOfInertia=[1 1 1]  MomentsOfInertiaUnits=kg*m^2  GraphicOpacity=viz.d2.palmar_interossei.spool_opacity  ProductsOfInertia=[0 0 0]  ProductsOfInertiaUnits=kg*m^2  GraphicShininess=75  GraphicSpecularColor=[0.5 0.5 0.5 1.0]  GraphicVisPropType=SimpleVisualProperties
  Tendon End : sm_lib/Belts and Cables/Belt-Cable End
      settings: SourceProductBaseCode=MS
  Tendon Spool : sm_lib/Belts and Cables/Belt-Cable Spool  PitchRadius=knm.d2.palmar_interossei.pitch_radius  PitchRadiusUnits=m  SenseSpoolAngleA=off  SenseFleetAngleA=off
      settings: SourceProductBaseCode=MS
  Insertion Point : PMIOPort  Side=Left
  Metacarpal Head Wrap : PMIOPort  Port=2  Side=Left
  Origin Point : PMIOPort  Port=3  Side=Left
  wires:
  Torque/1 -> Simulink-PS Converter/1
  connections:
  Revolute Joint1/LConn2 -- Simulink-PS Converter/RConn1
  Metacarpal Head Wrap Viz/RConn1 -- Metacarpal Head/LConn1 -- Revolute Joint2/RConn1
  Spool Viz/RConn1 -- Revolute Joint1/RConn1 -- Tendon Spool/LConn1
  Revolute Joint1/LConn1 -- Origin Point/RConn1
  Revolute Joint2/LConn1 -- Metacarpal Head Wrap/RConn1
  Insertion Point Viz/RConn1 -- Insertion Point/RConn1 -- Tendon End/LConn1
  Metacarpal Head/RConn1 -- Tendon End/RConn1
  Metacarpal Head/RConn2 -- Tendon Spool/RConn1 -- Belt-Cable Properties/LConn1
